simulink subsystem "Discrette_TF_Regulator"  (R2023a)
settings: Solver=VariableStepAuto  StartTime=0.0  StopTime=10.0  RelTol=1e-3
settings Model: Creator=user  LastModifiedBy=user

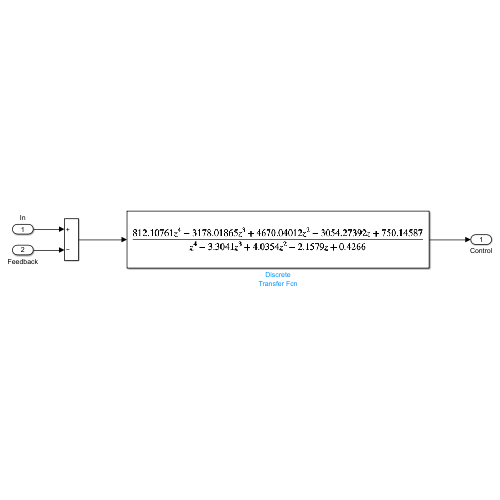
[thumbnail: Simulink's stored preview of the top-level diagram]
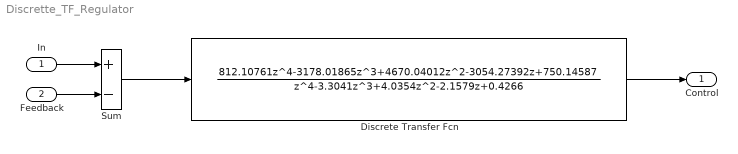
== system Discrette_TF_Regulator ==
  In : Inport
  Feedback : Inport  Port=2
  Discrete Transfer Fcn : DiscreteTransferFcn  Numerator=[812.10761, -3178.01865, 4670.04012, -3054.27392, 750.14587 ]  Denominator=[1, -3.3041, 4.0354, -2.1579, 0.4266]  SampleTime=0.005
  Sum : Sum  Inputs=+-
  Control : Outport
  wires:
  In/1 -> Sum/1
  Feedback/1 -> Sum/2
  Sum/1 -> Discrete Transfer Fcn/1
  Discrete Transfer Fcn/1 -> Control/1
